simulink model "DC_Motor_Model"  (R2022b)
settings: Solver=VariableStepAuto  StartTime=0.0  StopTime=10  RelTol=1e-3
values from neighbouring files (symbols this model uses):
  b = 10750    [DC_Motor_Parameters.m]
  J = 0.577e-2    (= 0.00577)    [DC_Motor_Parameters.m]
  Ke = 0.12    [DC_Motor_Parameters.m]
  Kt = 0.25    [DC_Motor_Parameters.m]
  L = 493e-9    (= 4.93e-07)    [DC_Motor_Parameters.m]
  R = 5.3e-3    (= 0.0053)    [DC_Motor_Parameters.m]
  T = 4.093 * (10^(-5))    (= 4.093e-05)    [DC_Motor_Parameters.m]    (also in Z_Domain_Parameters.m)
settings Model: Creator=frz  LastModifiedBy=frz

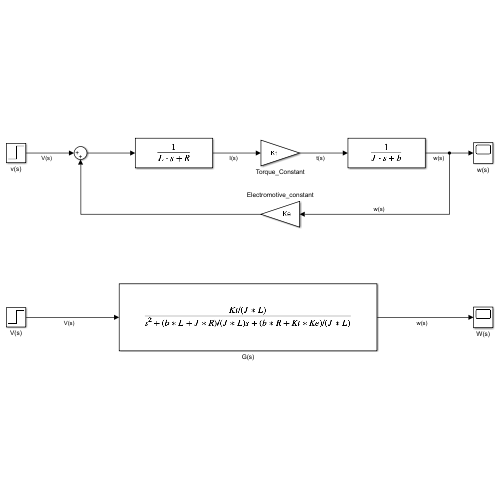
[thumbnail: Simulink's stored preview of the top-level diagram]
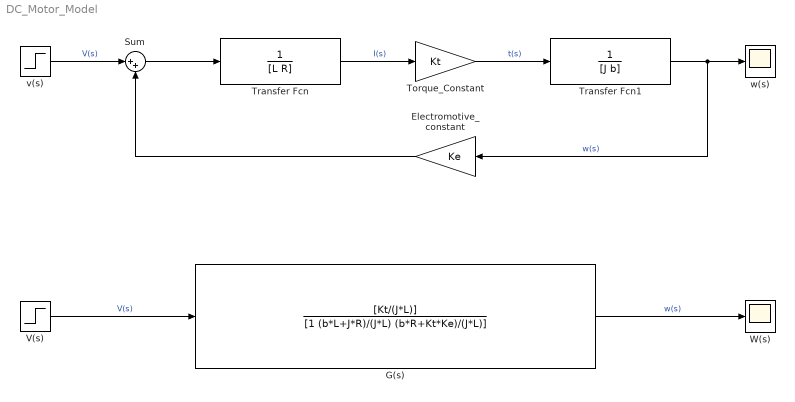
== system DC_Motor_Model ==
  Electromotive_constant : Gain  Gain=Ke
  G(s) : TransferFcn  Numerator=[Kt/(J*L)]  Denominator=[1 (b*L+J*R)/(J*L) (b*R+Kt*Ke)/(J*L)]
  Sum : Sum  Inputs=|++
  Torque_Constant : Gain  Gain=Kt
  Transfer Fcn : TransferFcn  Denominator=[L R]
  Transfer Fcn1 : TransferFcn  Denominator=[J b]
  V(s) : Step  Time=T  After=346  SampleTime=T
  W(s) : Scope
  v(s) : Step  Time=T  After=346  SampleTime=T
  w(s) : Scope
  wires:
  v(s)/1 -> Sum/1  "V(s)"
  Sum/1 -> Transfer Fcn/1
  Electromotive_constant/1 -> Sum/2
  Transfer Fcn/1 -> Torque_Constant/1  "I(s)"
  Torque_Constant/1 -> Transfer Fcn1/1  "t(s)"
  Transfer Fcn1/1 -> Electromotive_constant/1, w(s)/1  "w(s)"
  V(s)/1 -> G(s)/1  "V(s)"
  G(s)/1 -> W(s)/1  "w(s)"
